simulink model "program_counter2"  (R2020a)
settings: Solver=VariableStepAuto  StartTime=0.0  StopTime=inf  RelTol=1e-3
libraries: simulink_extras x5
settings Model: Creator=F1  LastModifiedBy=F1

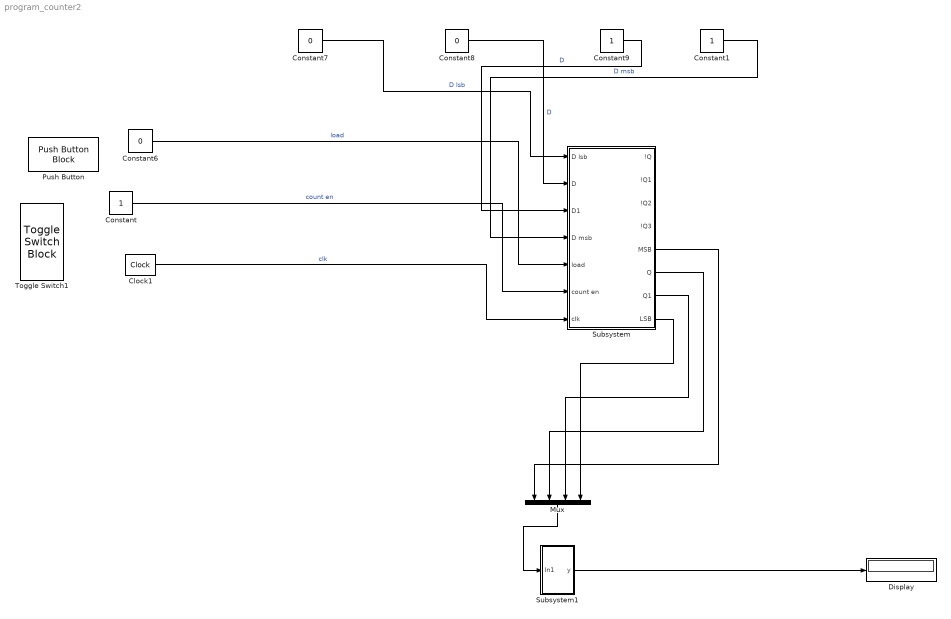
== system program_counter2 ==
  Clock1 : simulink_extras/Flip Flops/Clock  period=2
  Constant : Constant  OutDataTypeStr=boolean
  Constant1 : Constant
  Constant6 : Constant  Value=0  OutDataTypeStr=boolean
  Constant7 : Constant  Value=0
  Constant8 : Constant  Value=0
  Constant9 : Constant
  Display : Display
  Mux : Mux
  Push Button : PushButtonBlock
  Subsystem : Subsystem
  Subsystem1 : Subsystem
  Toggle Switch1 : ToggleSwitchBlock
      settings: Values={{'Off', 'On'}, [0 1]}
  wires:
  Subsystem1/1(y) -> Display/1
  Mux/1 -> Subsystem1/1(In1)
  Constant7/1 -> Subsystem/1(D lsb)  "D lsb"
  Constant8/1 -> Subsystem/2(D)  "D"
  Constant9/1 -> Subsystem/3(D1)  "D"
  Constant1/1 -> Subsystem/4(D msb)  "D msb"
  Constant6/1 -> Subsystem/5(load)  "load"
  Constant/1 -> Subsystem/6(count en)  "count en"
  Clock1/1 -> Subsystem/7(clk)  "clk"
  Subsystem/5(MSB) -> Mux/1
  Subsystem/6(Q) -> Mux/2
  Subsystem/7(Q1) -> Mux/3
  Subsystem/8(LSB) -> Mux/4

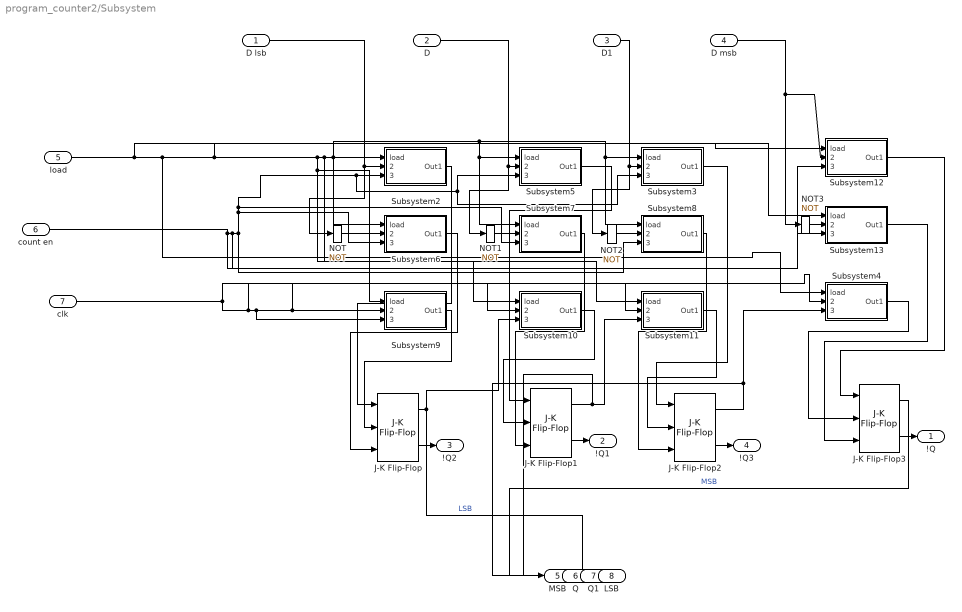
== system program_counter2/Subsystem ==
  D lsb : Inport
  D : Inport  Port=2
  D1 : Inport  Port=3
  D msb : Inport  Port=4
  load : Inport  Port=5
  count en : Inport  Port=6
  clk : Inport  Port=7
  J-K Flip-Flop{,1..3} (4 alike) : simulink_extras/Flip Flops/J-K Flip-Flop  initial_condition=0
  NOT{,1..3} (4 alike) : Logic  Operator=NOT  IconShape=distinctive  AllPortsSameDT=off  OutDataTypeStr=boolean
  Subsystem10 : Subsystem
  Subsystem11 : Subsystem
  Subsystem12 : Subsystem
  Subsystem13 : Subsystem
  Subsystem2 : Subsystem
  Subsystem3 : Subsystem
  Subsystem4 : Subsystem
  Subsystem5 : Subsystem
  Subsystem6 : Subsystem
  Subsystem7 : Subsystem
  Subsystem8 : Subsystem
  Subsystem9 : Subsystem
  !Q : Outport
  !Q1 : Outport  Port=2
  !Q2 : Outport  Port=3
  !Q3 : Outport  Port=4
  MSB : Outport  Port=5
  Q : Outport  Port=6
  Q1 : Outport  Port=7
  LSB : Outport  Port=8
  wires:
  count en/1 -> Subsystem12/3(select low), Subsystem13/3(select low), Subsystem5/3(select low), Subsystem3/3(select low), Subsystem2/3(select low), Subsystem7/3(select low), Subsystem6/3(select low), Subsystem8/3(select low)
  clk/1 -> Subsystem11/2(select high), Subsystem9/3(select low), Subsystem4/2(select high), Subsystem9/2(select high), Subsystem10/2(select high)
  Subsystem4/1(Out1) -> J-K Flip-Flop3/2
  Subsystem9/1(Out1) -> J-K Flip-Flop/2
  NOT2/1 -> Subsystem8/2(select high)
  Subsystem13/1(Out1) -> J-K Flip-Flop3/3
  load/1 -> Subsystem13/1(load), Subsystem4/1(load), Subsystem12/1(load), Subsystem10/1(load), Subsystem9/1(load), Subsystem11/1(load), Subsystem7/1(load), Subsystem5/1(load), Subsystem8/1(load), Subsystem3/1(load), Subsystem2/1(load), Subsystem6/1(load)
  J-K Flip-Flop3/2 -> !Q/1
  J-K Flip-Flop3/1 -> MSB/1  "MSB"
  Subsystem2/1(Out1) -> J-K Flip-Flop/1
  Subsystem12/1(Out1) -> J-K Flip-Flop3/1
  NOT/1 -> Subsystem6/2(select high)
  D/1 -> NOT1/1, Subsystem5/2(select high)
  Subsystem3/1(Out1) -> J-K Flip-Flop2/1
  NOT1/1 -> Subsystem7/2(select high)
  D msb/1 -> NOT3/1, Subsystem12/2(select high)
  Subsystem6/1(Out1) -> J-K Flip-Flop/3
  D lsb/1 -> NOT/1, Subsystem2/2(select high)
  Subsystem8/1(Out1) -> J-K Flip-Flop2/3
  NOT3/1 -> Subsystem13/2(select high)
  Subsystem10/1(Out1) -> J-K Flip-Flop1/2
  Subsystem5/1(Out1) -> J-K Flip-Flop1/1
  J-K Flip-Flop/1 -> LSB/1, Subsystem10/3(select low)  "LSB"
  D1/1 -> NOT2/1, Subsystem3/2(select high)
  J-K Flip-Flop1/2 -> !Q1/1
  Subsystem7/1(Out1) -> J-K Flip-Flop1/3
  J-K Flip-Flop1/1 -> Q1/1, Subsystem11/3(select low)
  J-K Flip-Flop2/2 -> !Q3/1
  J-K Flip-Flop2/1 -> Q/1, Subsystem4/3(select low)
  Subsystem11/1(Out1) -> J-K Flip-Flop2/2
  J-K Flip-Flop/2 -> !Q2/1

== system program_counter2/Subsystem1 ==
  In1 : Inport
  Demux : Demux
  MATLAB Function : MATLAB Function  TreatAsAtomicUnit=on
  y : Outport
  wires:
  Demux/3 -> MATLAB Function/3(b1)
  Demux/1 -> MATLAB Function/1(b3)
  Demux/2 -> MATLAB Function/2(b2)
  Demux/4 -> MATLAB Function/4(b0)
  MATLAB Function/1(y) -> y/1
  In1/1 -> Demux/1

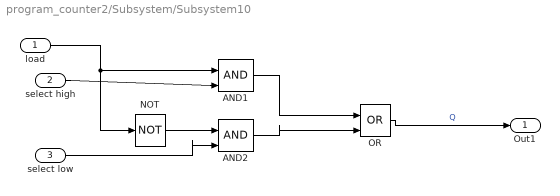
== system program_counter2/Subsystem/Subsystem10 ==
  load : Inport
  select high : Inport  Port=2
  select low : Inport  Port=3
  AND1 : Logic  IconShape=distinctive  AllPortsSameDT=off  OutDataTypeStr=boolean
  AND2 : Logic  IconShape=distinctive  AllPortsSameDT=off  OutDataTypeStr=boolean
  NOT : Logic  Operator=NOT  IconShape=distinctive  AllPortsSameDT=off  OutDataTypeStr=boolean
  OR : Logic  Operator=OR  IconShape=distinctive  AllPortsSameDT=off  OutDataTypeStr=boolean
  Out1 : Outport
  wires:
  select high/1 -> AND1/2
  OR/1 -> Out1/1  "Q"
  AND1/1 -> OR/1
  NOT/1 -> AND2/1
  AND2/1 -> OR/2
  load/1 -> NOT/1, AND1/1
  select low/1 -> AND2/2

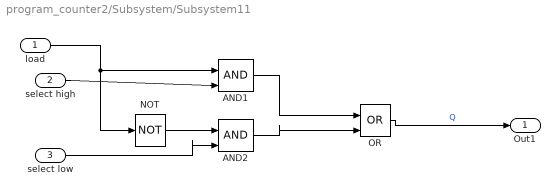
== system program_counter2/Subsystem/Subsystem11 ==
  load : Inport
  select high : Inport  Port=2
  select low : Inport  Port=3
  AND1 : Logic  IconShape=distinctive  AllPortsSameDT=off  OutDataTypeStr=boolean
  AND2 : Logic  IconShape=distinctive  AllPortsSameDT=off  OutDataTypeStr=boolean
  NOT : Logic  Operator=NOT  IconShape=distinctive  AllPortsSameDT=off  OutDataTypeStr=boolean
  OR : Logic  Operator=OR  IconShape=distinctive  AllPortsSameDT=off  OutDataTypeStr=boolean
  Out1 : Outport
  wires:
  select high/1 -> AND1/2
  OR/1 -> Out1/1  "Q"
  AND1/1 -> OR/1
  NOT/1 -> AND2/1
  AND2/1 -> OR/2
  load/1 -> NOT/1, AND1/1
  select low/1 -> AND2/2

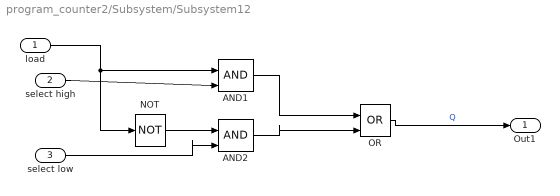
== system program_counter2/Subsystem/Subsystem12 ==
  load : Inport
  select high : Inport  Port=2
  select low : Inport  Port=3
  AND1 : Logic  IconShape=distinctive  AllPortsSameDT=off  OutDataTypeStr=boolean
  AND2 : Logic  IconShape=distinctive  AllPortsSameDT=off  OutDataTypeStr=boolean
  NOT : Logic  Operator=NOT  IconShape=distinctive  AllPortsSameDT=off  OutDataTypeStr=boolean
  OR : Logic  Operator=OR  IconShape=distinctive  AllPortsSameDT=off  OutDataTypeStr=boolean
  Out1 : Outport
  wires:
  select high/1 -> AND1/2
  OR/1 -> Out1/1  "Q"
  AND1/1 -> OR/1
  NOT/1 -> AND2/1
  AND2/1 -> OR/2
  load/1 -> NOT/1, AND1/1
  select low/1 -> AND2/2

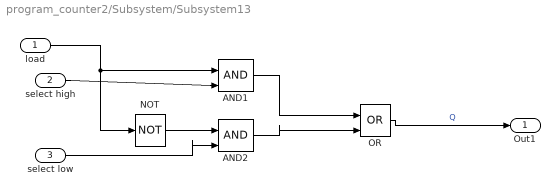
== system program_counter2/Subsystem/Subsystem13 ==
  load : Inport
  select high : Inport  Port=2
  select low : Inport  Port=3
  AND1 : Logic  IconShape=distinctive  AllPortsSameDT=off  OutDataTypeStr=boolean
  AND2 : Logic  IconShape=distinctive  AllPortsSameDT=off  OutDataTypeStr=boolean
  NOT : Logic  Operator=NOT  IconShape=distinctive  AllPortsSameDT=off  OutDataTypeStr=boolean
  OR : Logic  Operator=OR  IconShape=distinctive  AllPortsSameDT=off  OutDataTypeStr=boolean
  Out1 : Outport
  wires:
  select high/1 -> AND1/2
  OR/1 -> Out1/1  "Q"
  AND1/1 -> OR/1
  NOT/1 -> AND2/1
  AND2/1 -> OR/2
  load/1 -> NOT/1, AND1/1
  select low/1 -> AND2/2

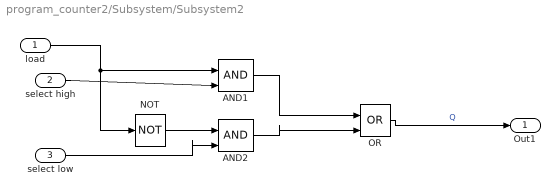
== system program_counter2/Subsystem/Subsystem2 ==
  load : Inport
  select high : Inport  Port=2
  select low : Inport  Port=3
  AND1 : Logic  IconShape=distinctive  AllPortsSameDT=off  OutDataTypeStr=boolean
  AND2 : Logic  IconShape=distinctive  AllPortsSameDT=off  OutDataTypeStr=boolean
  NOT : Logic  Operator=NOT  IconShape=distinctive  AllPortsSameDT=off  OutDataTypeStr=boolean
  OR : Logic  Operator=OR  IconShape=distinctive  AllPortsSameDT=off  OutDataTypeStr=boolean
  Out1 : Outport
  wires:
  select high/1 -> AND1/2
  OR/1 -> Out1/1  "Q"
  AND1/1 -> OR/1
  NOT/1 -> AND2/1
  AND2/1 -> OR/2
  load/1 -> NOT/1, AND1/1
  select low/1 -> AND2/2

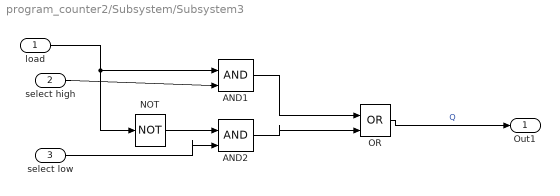
== system program_counter2/Subsystem/Subsystem3 ==
  load : Inport
  select high : Inport  Port=2
  select low : Inport  Port=3
  AND1 : Logic  IconShape=distinctive  AllPortsSameDT=off  OutDataTypeStr=boolean
  AND2 : Logic  IconShape=distinctive  AllPortsSameDT=off  OutDataTypeStr=boolean
  NOT : Logic  Operator=NOT  IconShape=distinctive  AllPortsSameDT=off  OutDataTypeStr=boolean
  OR : Logic  Operator=OR  IconShape=distinctive  AllPortsSameDT=off  OutDataTypeStr=boolean
  Out1 : Outport
  wires:
  select high/1 -> AND1/2
  OR/1 -> Out1/1  "Q"
  AND1/1 -> OR/1
  NOT/1 -> AND2/1
  AND2/1 -> OR/2
  load/1 -> NOT/1, AND1/1
  select low/1 -> AND2/2

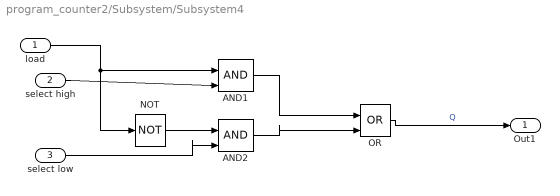
== system program_counter2/Subsystem/Subsystem4 ==
  load : Inport
  select high : Inport  Port=2
  select low : Inport  Port=3
  AND1 : Logic  IconShape=distinctive  AllPortsSameDT=off  OutDataTypeStr=boolean
  AND2 : Logic  IconShape=distinctive  AllPortsSameDT=off  OutDataTypeStr=boolean
  NOT : Logic  Operator=NOT  IconShape=distinctive  AllPortsSameDT=off  OutDataTypeStr=boolean
  OR : Logic  Operator=OR  IconShape=distinctive  AllPortsSameDT=off  OutDataTypeStr=boolean
  Out1 : Outport
  wires:
  select high/1 -> AND1/2
  OR/1 -> Out1/1  "Q"
  AND1/1 -> OR/1
  NOT/1 -> AND2/1
  AND2/1 -> OR/2
  load/1 -> NOT/1, AND1/1
  select low/1 -> AND2/2

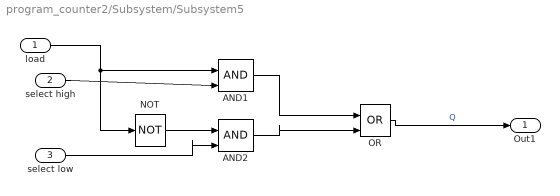
== system program_counter2/Subsystem/Subsystem5 ==
  load : Inport
  select high : Inport  Port=2
  select low : Inport  Port=3
  AND1 : Logic  IconShape=distinctive  AllPortsSameDT=off  OutDataTypeStr=boolean
  AND2 : Logic  IconShape=distinctive  AllPortsSameDT=off  OutDataTypeStr=boolean
  NOT : Logic  Operator=NOT  IconShape=distinctive  AllPortsSameDT=off  OutDataTypeStr=boolean
  OR : Logic  Operator=OR  IconShape=distinctive  AllPortsSameDT=off  OutDataTypeStr=boolean
  Out1 : Outport
  wires:
  select high/1 -> AND1/2
  OR/1 -> Out1/1  "Q"
  AND1/1 -> OR/1
  NOT/1 -> AND2/1
  AND2/1 -> OR/2
  load/1 -> NOT/1, AND1/1
  select low/1 -> AND2/2

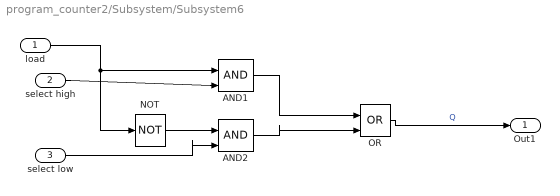
== system program_counter2/Subsystem/Subsystem6 ==
  load : Inport
  select high : Inport  Port=2
  select low : Inport  Port=3
  AND1 : Logic  IconShape=distinctive  AllPortsSameDT=off  OutDataTypeStr=boolean
  AND2 : Logic  IconShape=distinctive  AllPortsSameDT=off  OutDataTypeStr=boolean
  NOT : Logic  Operator=NOT  IconShape=distinctive  AllPortsSameDT=off  OutDataTypeStr=boolean
  OR : Logic  Operator=OR  IconShape=distinctive  AllPortsSameDT=off  OutDataTypeStr=boolean
  Out1 : Outport
  wires:
  select high/1 -> AND1/2
  OR/1 -> Out1/1  "Q"
  AND1/1 -> OR/1
  NOT/1 -> AND2/1
  AND2/1 -> OR/2
  load/1 -> NOT/1, AND1/1
  select low/1 -> AND2/2

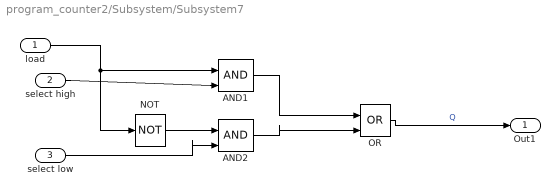
== system program_counter2/Subsystem/Subsystem7 ==
  load : Inport
  select high : Inport  Port=2
  select low : Inport  Port=3
  AND1 : Logic  IconShape=distinctive  AllPortsSameDT=off  OutDataTypeStr=boolean
  AND2 : Logic  IconShape=distinctive  AllPortsSameDT=off  OutDataTypeStr=boolean
  NOT : Logic  Operator=NOT  IconShape=distinctive  AllPortsSameDT=off  OutDataTypeStr=boolean
  OR : Logic  Operator=OR  IconShape=distinctive  AllPortsSameDT=off  OutDataTypeStr=boolean
  Out1 : Outport
  wires:
  select high/1 -> AND1/2
  OR/1 -> Out1/1  "Q"
  AND1/1 -> OR/1
  NOT/1 -> AND2/1
  AND2/1 -> OR/2
  load/1 -> NOT/1, AND1/1
  select low/1 -> AND2/2

== system program_counter2/Subsystem/Subsystem8 ==
  load : Inport
  select high : Inport  Port=2
  select low : Inport  Port=3
  AND1 : Logic  IconShape=distinctive  AllPortsSameDT=off  OutDataTypeStr=boolean
  AND2 : Logic  IconShape=distinctive  AllPortsSameDT=off  OutDataTypeStr=boolean
  NOT : Logic  Operator=NOT  IconShape=distinctive  AllPortsSameDT=off  OutDataTypeStr=boolean
  OR : Logic  Operator=OR  IconShape=distinctive  AllPortsSameDT=off  OutDataTypeStr=boolean
  Out1 : Outport
  wires:
  select high/1 -> AND1/2
  OR/1 -> Out1/1  "Q"
  AND1/1 -> OR/1
  NOT/1 -> AND2/1
  AND2/1 -> OR/2
  load/1 -> NOT/1, AND1/1
  select low/1 -> AND2/2

== system program_counter2/Subsystem/Subsystem9 ==
  load : Inport
  select high : Inport  Port=2
  select low : Inport  Port=3
  AND1 : Logic  IconShape=distinctive  AllPortsSameDT=off  OutDataTypeStr=boolean
  AND2 : Logic  IconShape=distinctive  AllPortsSameDT=off  OutDataTypeStr=boolean
  NOT : Logic  Operator=NOT  IconShape=distinctive  AllPortsSameDT=off  OutDataTypeStr=boolean
  OR : Logic  Operator=OR  IconShape=distinctive  AllPortsSameDT=off  OutDataTypeStr=boolean
  Out1 : Outport
  wires:
  select high/1 -> AND1/2
  OR/1 -> Out1/1  "Q"
  AND1/1 -> OR/1
  NOT/1 -> AND2/1
  AND2/1 -> OR/2
  load/1 -> NOT/1, AND1/1
  select low/1 -> AND2/2

== matlab function program_counter2/Subsystem1/MATLAB Function ==
  data: b3 input; y output; b2 input; b1 input; b0 input
function y = fcn( b3   , b2   , b1    , b0    )
y =  b3*2^3 + b2*2^2 + b1*2^1 + b0*2^0 ;
end
